simulink model "valid"  (R2020b)
settings: Solver=VariableStepAuto  StartTime=0.0  StopTime=10  RelTol=1e-3
values from neighbouring files (symbols this model uses):
  kd = kpid.kd    [function_params.m]
  ki = kpid.ki    [function_params.m]
  kp = kpid.kp    [function_params.m]
  T = 1/(5*max(abs(p{1})))    [projetoPID.m]
  umax = 14    [function_params.m]
  umin = 0    [function_params.m]
undefined symbols (not defined in the file or in its folder): bm1, bm2, bp0, bp1, C, g, Jm, Jp, kaphi, ku1, ku2, ku3, ku4, l, La, m, Ra
settings Model: Creator=Erick  LastModifiedBy=Erick

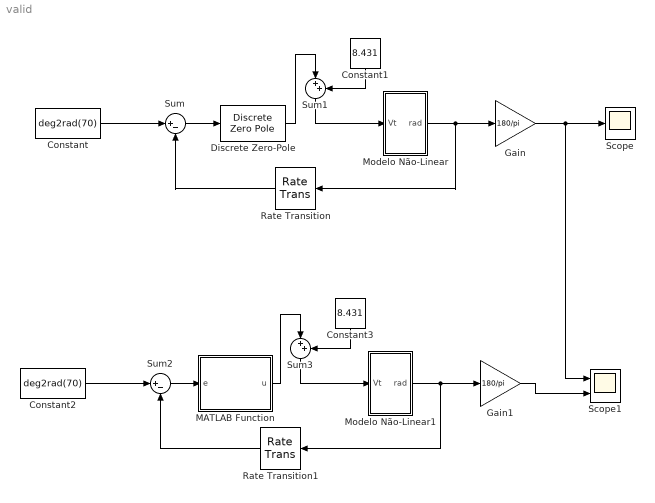
== system valid ==
  Constant : Constant  Value=deg2rad(70)
  Constant1 : Constant  Value=8.431
  Constant2 : Constant  Value=deg2rad(70)
  Constant3 : Constant  Value=8.431
  Discrete Zero-Pole : DiscreteZeroPole  Zeros=C.z{1}  Poles=C.p{1}  Gain=C.k  SampleTime=T
  Gain : Gain  Gain=180/pi
  Gain1 : Gain  Gain=180/pi
  MATLAB Function : MATLAB Function  TreatAsAtomicUnit=on
  Modelo Não-Linear : Subsystem
  Modelo Não-Linear1 : Subsystem
  Rate Transition : RateTransition  OutPortSampleTime=T
  Rate Transition1 : RateTransition  OutPortSampleTime=T
  Scope : Scope
  Scope1 : Scope  NumInputPorts=2
  Sum : Sum  Inputs=|+-
  Sum1 : Sum  Inputs=|++
  Sum2 : Sum  Inputs=|+-
  Sum3 : Sum  Inputs=|++
  wires:
  Sum/1 -> Discrete Zero-Pole/1
  Modelo Não-Linear/1(rad) -> Gain/1, Rate Transition/1
  Gain/1 -> Scope1/1, Scope/1
  Rate Transition/1 -> Sum/2
  Constant/1 -> Sum/1
  Discrete Zero-Pole/1 -> Sum1/1
  Sum1/1 -> Modelo Não-Linear/1(Vt)
  Constant1/1 -> Sum1/2
  Modelo Não-Linear1/1(rad) -> Gain1/1, Rate Transition1/1
  Sum3/1 -> Modelo Não-Linear1/1(Vt)
  Constant3/1 -> Sum3/2
  Constant2/1 -> Sum2/1
  Gain1/1 -> Scope1/2
  Rate Transition1/1 -> Sum2/2
  Sum2/1 -> MATLAB Function/1(e)
  MATLAB Function/1(u) -> Sum3/1

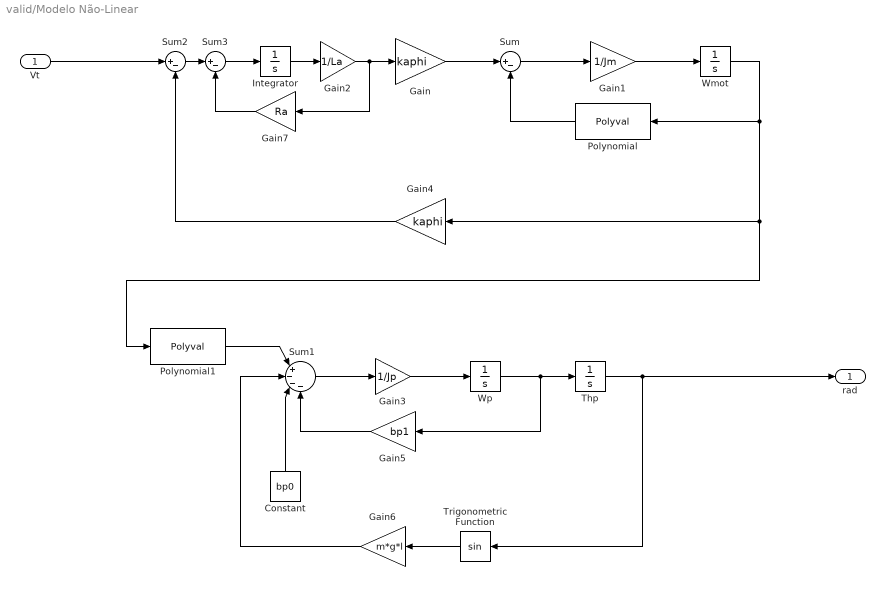
== system valid/Modelo Não-Linear ==
  Vt : Inport
  Constant : Constant  Value=bp0
  Gain : Gain  Gain=kaphi
  Gain1 : Gain  Gain=1/Jm
  Gain2 : Gain  Gain=1/La
  Gain3 : Gain  Gain=1/Jp
  Gain4 : Gain  Gain=kaphi
  Gain5 : Gain  Gain=bp1
  Gain6 : Gain  Gain=m*g*l
  Gain7 : Gain  Gain=Ra
  Integrator : Integrator  InitialCondition=1.867e-3
  Polynomial : Polyval  Coefs=[bm2, bm1, 0]
  Polynomial1 : Polyval  Coefs=[ku4, ku3, ku2, ku1, 0]
  Sum : Sum  Inputs=|+-
  Sum1 : Sum  Inputs=|+---
  Sum2 : Sum  Inputs=|+-
  Sum3 : Sum  Inputs=|+-
  Thp : Integrator  InitialCondition=0.8727  LimitOutput=on  UpperSaturationLimit=deg2rad(90)  LowerSaturationLimit=0
  Trigonometric Function : Trigonometry
  Wmot : Integrator  InitialCondition=372.2
  Wp : Integrator
  rad : Outport
  wires:
  Constant/1 -> Sum1/3
  Wmot/1 -> Polynomial1/1, Gain4/1, Polynomial/1
  Sum/1 -> Gain1/1
  Trigonometric Function/1 -> Gain6/1
  Gain1/1 -> Wmot/1
  Polynomial/1 -> Sum/2
  Gain4/1 -> Sum2/2
  Vt/1 -> Sum2/1
  Thp/1 -> rad/1, Trigonometric Function/1
  Gain/1 -> Sum/1
  Gain6/1 -> Sum1/2
  Wp/1 -> Gain5/1, Thp/1
  Sum1/1 -> Gain3/1
  Gain5/1 -> Sum1/4
  Gain3/1 -> Wp/1
  Polynomial1/1 -> Sum1/1
  Sum2/1 -> Sum3/1
  Sum3/1 -> Integrator/1
  Integrator/1 -> Gain2/1
  Gain2/1 -> Gain7/1, Gain/1
  Gain7/1 -> Sum3/2

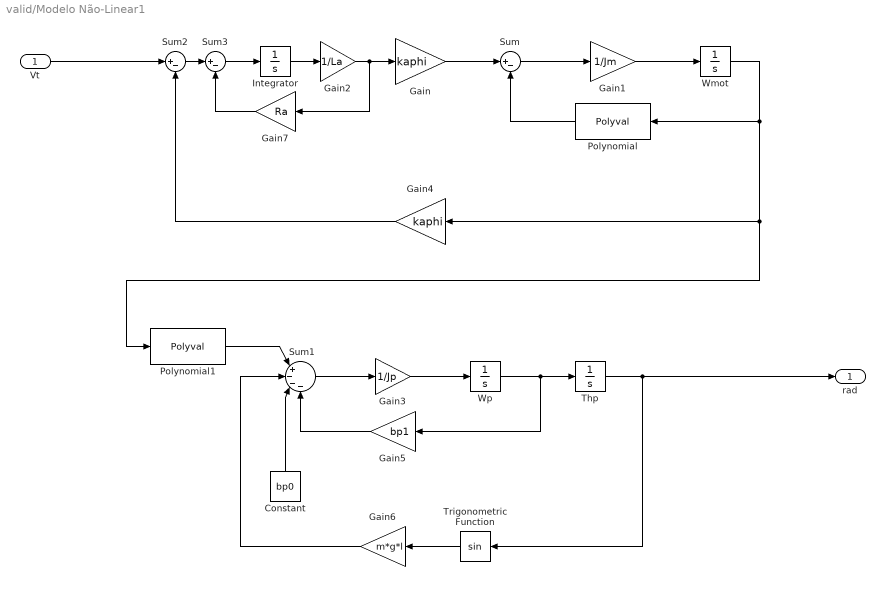
== system valid/Modelo Não-Linear1 ==
  Vt : Inport
  Constant : Constant  Value=bp0
  Gain : Gain  Gain=kaphi
  Gain1 : Gain  Gain=1/Jm
  Gain2 : Gain  Gain=1/La
  Gain3 : Gain  Gain=1/Jp
  Gain4 : Gain  Gain=kaphi
  Gain5 : Gain  Gain=bp1
  Gain6 : Gain  Gain=m*g*l
  Gain7 : Gain  Gain=Ra
  Integrator : Integrator  InitialCondition=1.867e-3
  Polynomial : Polyval  Coefs=[bm2, bm1, 0]
  Polynomial1 : Polyval  Coefs=[ku4, ku3, ku2, ku1, 0]
  Sum : Sum  Inputs=|+-
  Sum1 : Sum  Inputs=|+---
  Sum2 : Sum  Inputs=|+-
  Sum3 : Sum  Inputs=|+-
  Thp : Integrator  InitialCondition=0.8727  LimitOutput=on  UpperSaturationLimit=deg2rad(90)  LowerSaturationLimit=0
  Trigonometric Function : Trigonometry
  Wmot : Integrator  InitialCondition=372.2
  Wp : Integrator
  rad : Outport
  wires:
  Constant/1 -> Sum1/3
  Wmot/1 -> Polynomial1/1, Gain4/1, Polynomial/1
  Sum/1 -> Gain1/1
  Trigonometric Function/1 -> Gain6/1
  Gain1/1 -> Wmot/1
  Polynomial/1 -> Sum/2
  Gain4/1 -> Sum2/2
  Vt/1 -> Sum2/1
  Thp/1 -> rad/1, Trigonometric Function/1
  Gain/1 -> Sum/1
  Gain6/1 -> Sum1/2
  Wp/1 -> Gain5/1, Thp/1
  Sum1/1 -> Gain3/1
  Gain5/1 -> Sum1/4
  Gain3/1 -> Wp/1
  Polynomial1/1 -> Sum1/1
  Sum2/1 -> Sum3/1
  Sum3/1 -> Integrator/1
  Integrator/1 -> Gain2/1
  Gain2/1 -> Gain7/1, Gain/1
  Gain7/1 -> Sum3/2

== matlab function valid/MATLAB Function ==
  data: e input; u output; kp parameter; ki parameter; kd parameter; T parameter; umax parameter; umin parameter
function u = meu_pid(e, kp, ki, kd, T, umax, umin)
    persistent ea;
    persistent uia;
    if (isempty(ea))
        ea = 0;
        uia = 0;
    end
    duia = ki*T*e;
    ud = (e - ea)*kd/T;

    u = kp*e + ud + uia + duia;
    ea = e;

    if (u > umax)
        u = umax;
    else if (u < umin)
        u = umin;
        else
        uia = uia + duia;
    end
    end
end
